simulink model "auv_simulink"  (R2021b)
settings: Solver=VariableStepAuto  StartTime=0.0  StopTime=60  RelTol=1e-3
undefined symbols (not defined in the file): B, D_LIN, D_QUAD, I0, m, M_A, r_b_b, r_g_b, tau_c
libraries: slpidlib x4
settings Model: Creator=User  LastModifiedBy=User

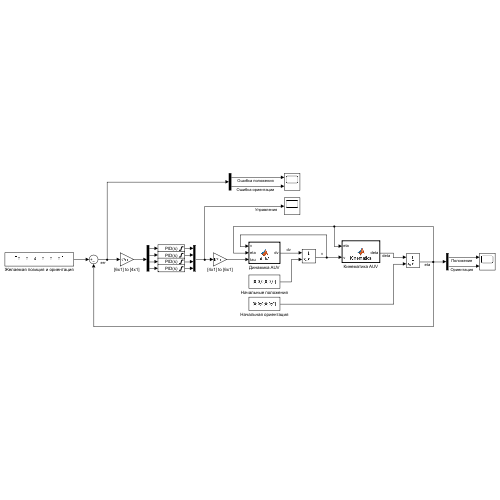
[thumbnail: Simulink's stored preview of the top-level diagram]
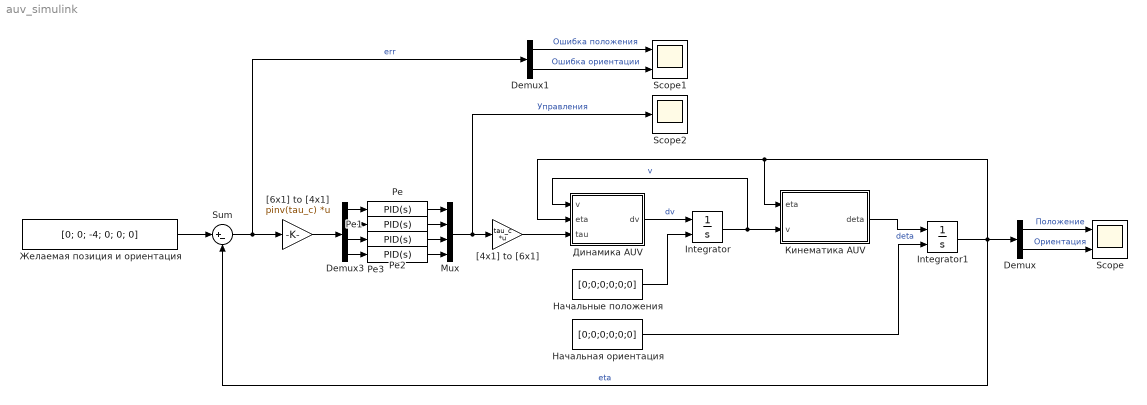
== system auv_simulink ==
  Demux : Demux  Outputs=2
  Demux1 : Demux  Outputs=2
  Demux3 : Demux
  Integrator : Integrator  InitialConditionSource=external  UpperSaturationLimit=1000  LowerSaturationLimit=-1000
  Integrator1 : Integrator  InitialConditionSource=external  UpperSaturationLimit=1000  LowerSaturationLimit=-1000
  Mux : Mux
  Scope : Scope  NumInputPorts=2
  Scope1 : Scope  NumInputPorts=2
  Scope2 : Scope
  Sum : Sum  Inputs=|+-
  "[4x1] to [6x1]" : Gain  Gain=tau_c  Multiplication=Matrix(K*u)
  "[6x1] to [4x1]" : Gain  Gain=pinv(tau_c)  Multiplication=Matrix(K*u)
  Динамика AUV : MATLAB Function  TreatAsAtomicUnit=on
  Желаемая позиция и ориентация : Constant  Value=[0; 0; -4; 0; 0; 0]
  Кинематика AUV : MATLAB Function  TreatAsAtomicUnit=on
  Начальная ориентация : Constant  Value=[0;0;0;0;0;0]
  Начальные положения : Constant  Value=[0;0;0;0;0;0]
  Ре{,1..3} (4 alike) : slpidlib/PID Controller  Controller=PID  Form=Parallel  TimeDomain=Continuous-time  UseExternalTs=off  SampleTime=-1  IntegratorMethod=Forward Euler  FilterMethod=Forward Euler  ControllerParametersSource=internal  P=4  I=0.3  D=1.8  UseFilter=on  N=100  TunerSelectOption=Transfer Function Based (PID Tuner App)  InitialConditionSource=internal  InitialConditionForIntegrator=0  InitialConditionForFilter=0  DifferentiatorICPrevScaledInput=0  ExternalReset=none  TrackingMode=off  Kt=1  LimitOutput=on  SatLimitsSource=internal  UpperSaturationLimit=1  LowerSaturationLimit=-1  LinearizeAsGain=on  AntiWindupMode=none  Kb=1  POutMin=[]  POutMax=[]  IOutMin=[]  IOutMax=[]  DOutMin=[]  DOutMax=[]  NOutMin=[]  NOutMax=[]  SumOutMin=[]  SumOutMax=[]  SaturationOutMin=[]  SaturationOutMax=[]  PParamMin=[]  PParamMax=[]  IParamMin=[]  IParamMax=[]  DParamMin=[]  DParamMax=[]  NParamMin=[]  NParamMax=[]  KbParamMin=[]  KbParamMax=[]  KtParamMin=[]  KtParamMax=[]  KbOutMin=[]  KbOutMax=[]  KtOutMin=[]  KtOutMax=[]  IntegratorOutMin=[]  IntegratorOutMax=[]  FilterOutMin=[]  FilterOutMax=[]  SumI1OutMin=[]  SumI1OutMax=[]  SumI2OutMin=[]  SumI2OutMax=[]  SumI3OutMin=[]  SumI3OutMax=[]  SumI4OutMin=[]  SumI4OutMax=[]  SumDOutMin=[]  SumDOutMax=[]  DifferentiatorOutMin=[]  DifferentiatorOutMax=[]  FilterDiffOutCoefMin=[]  FilterDiffOutCoefMax=[]  ReciprocalOutMin=[]  ReciprocalOutMax=[]  SumDenOutMin=[]  SumDenOutMax=[]  SumNumOutMin=[]  SumNumOutMax=[]  DivideOutMin=[]  DivideOutMax=[]  UdiffTsProdOutMin=[]  UdiffTsProdOutMax=[]  NTsProdOutMin=[]  NTsProdOutMax=[]  UintegralTsProdOutMin=[]  UintegralTsProdOutMax=[]  UngainTsProdOutMin=[]  UngainTsProdOutMax=[]  IntegratorContinuousStateAttributes=''  IntegratorStateMustResolveToSignalObject=off  IntegratorRTWStateStorageClass=Auto  FilterContinuousStateAttributes=''  FilterStateMustResolveToSignalObject=off  FilterRTWStateStorageClass=Auto  ParallelPVariant=InternalParameters  IdealPVariant=Disabled  IVariant=InternalParameters  DVariant=InternalParameters  IntegratorVariant=Continuous  SatVariant=Enabled  AWVariant=Passthrough  PCopyVariant=Disabled  TRVariant=Disabled  FdbkBlocksVariant=Forward  IdealPFdbkVariant=Disabled  SatFdbkVariant=Disabled  DerivativeFilterVariant=ContFilter  NVariant=InternalParameters  NCopyVariant=Disabled  FilterICVariant=InternalICsFilter  IntegratorICVariant=InternalICs  ExternalResetVariant=Disabled  TRSumVariant=Passthrough  SumFdbkVariant=Disabled  SumVariant=Sum_PID  TsampFilterVariant=InternalTs  TsampNgainVariant=Passthrough  TsampIntegralVariant=Passthrough  ExternalSaturationOutDataTypeStr=Inherit: Same as second input
  wires:
  Динамика AUV/1(dv) -> Integrator/1  "dv"
  Начальные положения/1 -> Integrator/2
  Integrator/1 -> Кинематика AUV/2(v), Динамика AUV/1(v)  "v"
  Начальная ориентация/1 -> Integrator1/2
  Integrator1/1 -> Sum/2, Demux/1, Кинематика AUV/1(eta), Динамика AUV/2(eta)  "eta"
  Demux/1 -> Scope/1  "Положение"
  Demux/2 -> Scope/2  "Ориентация"
  Demux1/2 -> Scope1/2  "Ошибка ориентации"
  Demux1/1 -> Scope1/1  "Ошибка положения"
  Кинематика AUV/1(deta) -> Integrator1/1  "deta"
  "[4x1] to [6x1]"/1 -> Динамика AUV/3(tau)
  Demux3/1 -> Ре/1
  Demux3/2 -> Ре1/1
  Demux3/3 -> Ре2/1
  Demux3/4 -> Ре3/1
  Ре/1 -> Mux/1
  Ре1/1 -> Mux/2
  Ре2/1 -> Mux/3
  Ре3/1 -> Mux/4
  Mux/1 -> Scope2/1, "[4x1] to [6x1]"/1  "Управления"
  Желаемая позиция и ориентация/1 -> Sum/1
  Sum/1 -> Demux1/1, "[6x1] to [4x1]"/1  "err"
  "[6x1] to [4x1]"/1 -> Demux3/1

== matlab function auv_simulink/Кинематика AUV ==
  data: eta input size=6; v input size=6; deta output size=6
function deta = Kinematics(eta,v)

%% РАСЧЕТ ЯКОБИАНА
J_k_o = [ 1  0           -sin(eta(5)); ...
          0  cos(eta(4))  cos(eta(5))*sin(eta(4)); ...
          0 -sin(eta(4))  cos(eta(5))*cos(eta(4)) ];
R_I_B = [ cos(eta(6))*cos(eta(5))                                         sin(eta(6))*cos(eta(5))                                        -sin(eta(5)); ...
         -sin(eta(6))*cos(eta(4)) + cos(eta(6))*sin(eta(5))*sin(eta(4))   cos(eta(6))*cos(eta(4)) + sin(eta(6))*sin(eta(5))*sin(eta(4))   sin(eta(4))*cos(eta(5)); ...
          sin(eta(6))*sin(eta(4)) + cos(eta(6))*sin(eta(5))*cos(eta(4))  -cos(eta(6))*sin(eta(4)) + sin(eta(6))*sin(eta(5))*cos(eta(4))   cos(eta(4))*cos(eta(5))];
J = [ R_I_B    zeros(3); ...
      zeros(3) J_k_o  ];

deta = inv(J)*v;

== matlab function auv_simulink/Динамика AUV ==
  data: v input size=6; dv output size=6; eta input size=6; tau input size=6; m parameter; r_b_b parameter size=[3 1]; r_g_b parameter size=[3 1]; I0 parameter size=[3 3]; D_LIN parameter size=[6 6]; D_QUAD parameter size=[6 6]; M_A parameter size=[6 6]; B parameter size=1
function dv = AUV(v,eta,tau, m, r_b_b, r_g_b, I0, D_LIN, D_QUAD, M_A, B)
%% ВСПОМОГАТЕЛЬНЫЕ ФУНКЦИИ
% преобразование в кососимметричную матрицу
S = @(x)([ 0 -x(3) x(2); x(3) 0 -x(1); -x(2) x(1) 0 ]); 

%% РАСЧЕТ МАТРИЦЫ M
% расчет M_RB
M_RB = [ m*eye(3) -m*S(r_g_b); m*S(r_g_b) I0 ]; 
% расчет M
M = M_RB + M_A; 

%% РАСЧЕТ C(v)
% расчет C_RB(v)
%C_RB = @(v)([ zeros(3) -m*S(v(1:3)); -m*S(v(1:3)) -S(diag(I0).*v(4:end)) ]); 
C_RB = @(v)[ zeros(3)                           -m*S(v(1:3))-m*S(S(v(4:end))*r_g_b); ...
            -m*S(v(1:3))-m*S(S(v(4:end))*r_g_b)  m*S(S(v(1:3))*r_g_b)-S(I0*v(4:end)) ];
% расчет C_A(v)
diag_M_A = diag(M_A);
C_A = @(v)([ zeros(3) -S(diag_M_A(1:3).*v(1:3)); 
    -S(diag_M_A(1:3).*v(1:3)) -S(diag_M_A(4:end).*v(4:end))]);
% расчет C(v)
C = @(v)(C_RB(v) + C_A(v)); 
% M11 = M(1:3,1:3); M12 = M(1:3,4:6); M21 = M(4:6,1:3); M22 = M(4:6,4:6);
% C = @(v)[ zeros(3) -S(M11*v(1:3)+M12*v(4:6)); -S(M11*v(1:3)+M12*v(4:6)) -S(M21*v(1:3)+M22*v(4:6)) ];

%% РАСЧЕТ g(n)
x_g = r_g_b(1); y_g = r_g_b(2); z_g = r_g_b(3);
x_b = r_b_b(1); y_b = r_b_b(2); z_b = r_b_b(3);
g = @(eta)[ (m*9.81-B)*sin(eta(5)); 
           -(m*9.81-B)*cos(eta(5))*sin(eta(4)); 
           -(m*9.81-B)*cos(eta(5))*cos(eta(4));
           -(y_g*m*9.81-y_b*B)*cos(eta(5))*cos(eta(4)) + ...
              (z_g*m*9.81-z_b*B)*cos(eta(5))*sin(eta(4));
            (z_g*m*9.81-z_b*B)*sin(eta(5)) + ...
              (x_g*m*9.81-x_b*B)*cos(eta(5))*cos(eta(4));
           -(x_g*m*9.81-x_b*B)*cos(eta(5))*sin(eta(4)) - ...
              (y_g*m*9.81-y_b*B)*sin(eta(5)) ]; 

%% РАСЧЕТ D(v)
D = @(v)(D_LIN + D_QUAD.*abs(v));

dv = -M^-1 * ( ( C(v) + D(v) )*v + g(eta) - tau);
